simulink model "s4"  (Simulink 2.00)
settings: Solver=ode15s  StartTime=0.0  StopTime=tstop  MaxStep=0.1  RelTol=1e-6  AbsTol=1e-6
values from neighbouring files (symbols this model uses):
  AEx = 0.0012    [I3ESSR.M]    (also in SET1.M)
  BEx = 1.264    [I3ESSR.M]    (also in SET1.M)
  delio = x(3)    [M1.M]    (also in M3.M = delta4; M3G.M = delta4; M4.M = delta)
  Domega = 0    [I3ESSR.M]    (also in M3.M; M3G.M; M5.M = 1; SET1.M = 2)
  Dz = (rs+re)*(rs+re) + (xq+xe)*(xpd+xe)    [M1.M]    (also in M4.M = (re+rs)*(re+rs) + (xe + xq)*(xe + xpd))
  Edpo = x(2)    [M1.M]    (also in M4.M = Vdo - xpq*Iqo + rs*Ido)
  Efo = u(1)    [M1.M]    (also in M3.M = Eqo + (xd-xq)*Ido; M3G.M = Eqo + (xd-xq)*Ido; M4.M = Eqo + (xd-xq)*Ido)
  Eqpo = x(1)    [M1.M]    (also in M4.M = Vqo + xpd*Ido + rs*Iqo)
  H = 2.89    [I3ESSR.M]    (also in M1.M = 0.5*J_rotor*wbasem*wbasem/Sbase; M3.M = diag(h); M3G.M = diag(h); M5.M = 0.352825293175)
  KA = 50    [I3ESSR.M]    (also in SET1.M)
  KE = -0.0465    [I3ESSR.M]    (also in SET1.M)
  KF = 0.0832    [I3ESSR.M]    (also in SET1.M)
  Ks = 120    [M4.M]    (also in M4COMP.M)
  Pmecho = real(Sto)    [M4.M]
  pss_limit = 0.1    [M4.M]
  pss_sw = 5    [M4.M]
  re = 0.0    (= 0)    [M1.M]
  rs = 0.00    (= 0)    [I3ESSR.M]    (also in M1.M = rs/Zbase; M3.M; M3G.M = 0.001; M5.M = rs/Zb)
  T1 = 0.024    [M4.M]    (also in M4COMP.M)
  T2 = 0.002    [M4.M]    (also in M4COMP.M)
  T3 = 0.024    [M4.M]    (also in M4COMP.M)
  T4 = 0.24    [M4.M]    (also in M4COMP.M)
  TA = .06    (= 0.06)    [I3ESSR.M]    (also in SET1.M)
  TE = 0.052    [I3ESSR.M]    (also in SET1.M)
  TF = 1.0    (= 1)    [I3ESSR.M]    (also in SET1.M)
  Tpdo = 4.3    [I3ESSR.M]    (also in SET1.M = 7.9)
  Tpqo = 0.85    [I3ESSR.M]    (also in SET1.M = 0.41)
  Tw = 1.    (= 1)    [M4.M]    (also in M4COMP.M)
  Vio = abs(Vi)    [M4.M]
  VR = KE*Efo    [M4.M]
  Vref = abs(Vto)    [M4.M]
  VRmax = 1    [I3ESSR.M]    (also in SET1.M)
  VRmin = -1    [I3ESSR.M]    (also in SET1.M)
  Vs = Efo*KF/TF    [M4.M]
  wb = wbase    [M1.M]    (also in M2.M = 376.991118431; M3.M = 376.991118431; M3G.M = 376.991118431; M4.M = we)
  we = 2*pi*Frated    [M1.M]    (also in M4.M; M5.M = 710.48)
  xe = 0.0    (= 0)    [M1.M]    (also in M4.M = 0.1)
  xpd = 0.169    [I3ESSR.M]    (also in M1.M = xpd/Zbase; SET1.M = 0.355)
  xq = 1.71    [I3ESSR.M]    (also in M1.M = xq/Zbase; M3.M; M3G.M; M5.M = xq/Zb)
settings Model: SaveTime=off  SaveOutput=off  ConsistencyChecking=off

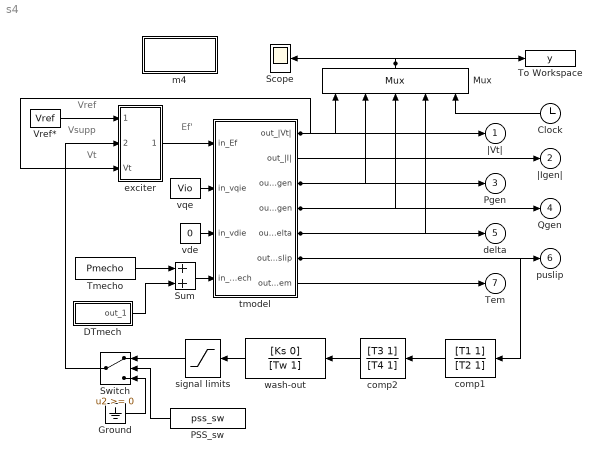
== system s4 ==
  note: Ef'
  note: Vsupp
  note: Vt
  note: Vref
  Clock : Clock
      settings: DeleteFcn=simclock BlockIsBeingDestroyed  PostSaveFcn=simclock Save
  DTmech : Subsystem  mask(Repeating table){@1=time_Dtmech, @2=tmech_Dtmech}
      mask prompts: @1 "Time values:"; @2 "Output values:"
      mask help:
      | Repeating table.
      | Enter values of time and output for first cycle.
      mask init:
      | period = max(@1); t = @1; y = @2;
      mask Help: Repeats cycle given in table. Time values should be monotonically increasing.
      mask Display: plot([t,t+period,t+2*period],[y,y,y])
  Ground : Ground
  m4 : Subsystem
      settings: OpenFcn=m4
      mask Type: Masked block of m4.m
      mask Help: Uses m4.m to initialize and plot
      mask Display: disp('Initialize\nand plot')
  Mux : Mux  Orientation=up  Inputs=5
  PSS_sw : Constant  Orientation=left  Value=pss_sw
  Scope : Scope
      settings: TickLabels=on  TimeRange=30  YMin=-2  YMax=2  SaveToWorkspace=off  SaveName=ScopeData  LimitMaxRows=off
  Sum : Sum  Inputs=++
  Switch : Switch  Orientation=left  Threshold=0
  Tmecho : Constant  Value=Pmecho
  To Workspace : ToWorkspace  VariableName=y  SampleTime=0
      settings: Buffer=10000
  Vref* : Constant  Value=Vref
  comp1 : TransferFcn  Orientation=left  Numerator=[T1 1]  Denominator=[T2 1]
  comp2 : TransferFcn  Orientation=left  Numerator=[T3 1]  Denominator=[T4 1]
  exciter : Subsystem
  signal limits : Saturate  Orientation=left  UpperLimit=pss_limit  LowerLimit=-pss_limit
  tmodel : Subsystem
  vde : Constant  Value=0
  vqe : Constant  Value=Vio
  wash-out : TransferFcn  Orientation=left  Numerator=[Ks 0]  Denominator=[Tw 1]
  |Vt| : Outport  Port=1  InitialOutput=0
  |Igen| : Outport  Port=2  InitialOutput=0
  Pgen : Outport  Port=3  InitialOutput=0
  Qgen : Outport  Port=4  InitialOutput=0
  delta : Outport  Port=5  InitialOutput=0
  puslip : Outport  Port=6  InitialOutput=0
  Tem : Outport  Port=7  InitialOutput=0
  wires:
  vqe/1 -> tmodel/2(in_vqie)
  vde/1 -> tmodel/3(in_vdie)
  tmodel/7(out_Tem) -> Tem/1
  tmodel/2(out_|I|) -> |Igen|/1
  Mux/1 -> Scope/1, To Workspace/1
  tmodel/1(out_|Vt|) -> |Vt|/1, Mux/1, exciter/3(Vt)
  exciter/1(out_Ef) -> tmodel/1(in_Ef)
  comp2/1 -> wash-out/1
  comp1/1 -> comp2/1
  tmodel/6(out_puslip) -> puslip/1, comp1/1
  wash-out/1 -> signal limits/1
  signal limits/1 -> Switch/1
  Switch/1 -> exciter/2(Vsupp)
  PSS_sw/1 -> Switch/2
  Vref*/1 -> exciter/1(Vref)
  Tmecho/1 -> Sum/1
  Sum/1 -> tmodel/4(in_Tmech)
  tmodel/3(out_Pgen) -> Pgen/1, Mux/2
  tmodel/4(out_Qgen) -> Qgen/1, Mux/3
  tmodel/5(out_delta) -> delta/1, Mux/4
  Clock/1 -> Mux/5
  DTmech/1(out_1) -> Sum/2
  Ground/1 -> Switch/3

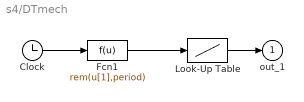
== system s4/DTmech ==
  Clock : Clock
      settings: DeleteFcn=simclock BlockIsBeingDestroyed  PostSaveFcn=simclock Save
  Fcn1 : Fcn  Expr=rem(u[1],period)
  Look-Up Table : Lookup  InputValues=t  OutputValues=y
  out_1 : Outport  Port=1  InitialOutput=0
  wires:
  Look-Up Table/1 -> out_1/1
  Clock/1 -> Fcn1/1
  Fcn1/1 -> Look-Up Table/1

== system s4/m4 ==
  note: Masked block of m4.m to initialize
      | s4.m in chapter 10 and to plot results

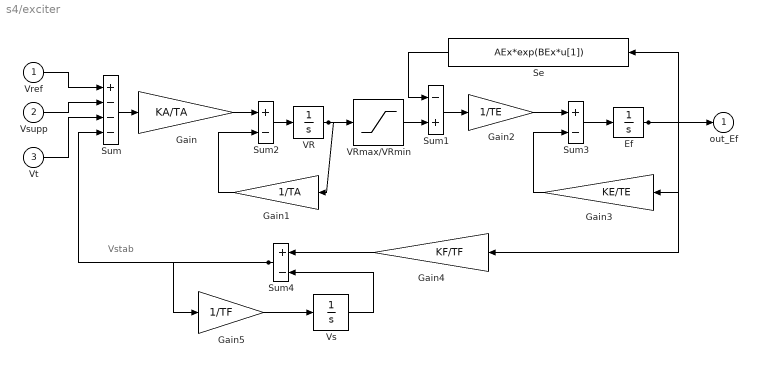
== system s4/exciter ==
  note: Vstab
  Vref : Inport  Port=1  PortWidth=-1  SampleTime=-1
  Vsupp : Inport  Port=2  PortWidth=-1  SampleTime=-1
  Vt : Inport  Port=3  PortWidth=-1  SampleTime=-1
  Ef : Integrator  ExternalReset=none  InitialConditionSource=internal  InitialCondition=Efo  LimitOutput=off  UpperSaturationLimit=inf  LowerSaturationLimit=-inf  ShowSaturationPort=off  ShowStatePort=off  AbsoluteTolerance=auto
  Gain : Gain  Gain=KA/TA
  Gain1 : Gain  Orientation=left  Gain=1/TA
  Gain2 : Gain  Gain=1/TE
  Gain3 : Gain  Orientation=left  Gain=KE/TE
  Gain4 : Gain  Orientation=left  Gain=KF/TF
  Gain5 : Gain  Gain=1/TF
  Se : Fcn  Orientation=left  Expr=AEx*exp(BEx*u[1])
  Sum : Sum  Inputs=+---
  Sum1 : Sum  Inputs=-+
  Sum2 : Sum  Inputs=+-
  Sum3 : Sum  Inputs=+-
  Sum4 : Sum  Orientation=left  Inputs=+-
  VR : Integrator  ExternalReset=none  InitialConditionSource=internal  InitialCondition=VR  LimitOutput=off  UpperSaturationLimit=inf  LowerSaturationLimit=-inf  ShowSaturationPort=off  ShowStatePort=off  AbsoluteTolerance=auto
  VRmax/VRmin : Saturate  UpperLimit=VRmax  LowerLimit=VRmin
  Vs : Integrator  ExternalReset=none  InitialConditionSource=internal  InitialCondition=Vs  LimitOutput=off  UpperSaturationLimit=inf  LowerSaturationLimit=-inf  ShowSaturationPort=off  ShowStatePort=off  AbsoluteTolerance=auto
  out_Ef : Outport  Port=1  InitialOutput=0
  wires:
  VRmax/VRmin/1 -> Sum1/2
  Vref/1 -> Sum/1
  Se/1 -> Sum1/1
  Sum2/1 -> VR/1
  Sum/1 -> Gain/1
  VR/1 -> VRmax/VRmin/1, Gain1/1
  Sum3/1 -> Ef/1
  Sum1/1 -> Gain2/1
  Gain2/1 -> Sum3/1
  Gain3/1 -> Sum3/2
  Ef/1 -> Gain3/1, Se/1, out_Ef/1, Gain4/1
  Gain/1 -> Sum2/1
  Gain1/1 -> Sum2/2
  Gain4/1 -> Sum4/1
  Gain5/1 -> Vs/1
  Vs/1 -> Sum4/2
  Sum4/1 -> Gain5/1, Sum/4
  Vt/1 -> Sum/3
  Vsupp/1 -> Sum/2

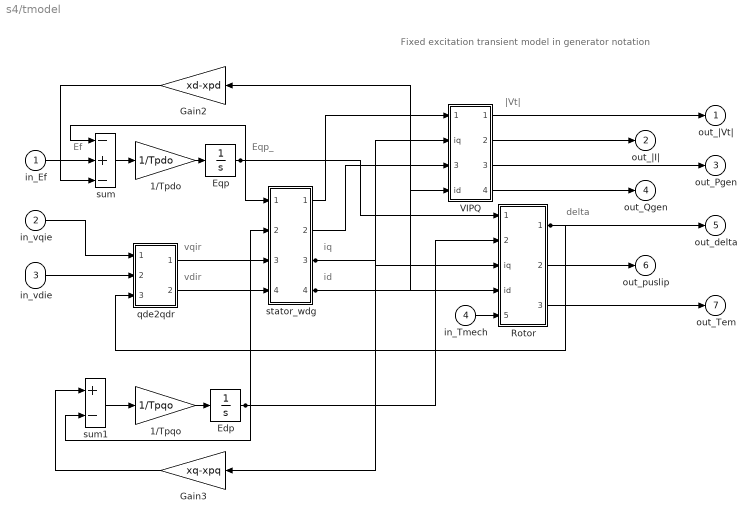
== system s4/tmodel ==
  note: Fixed excitation transient model in generator notation
  note: |Vt|
  note: id
  note: iq
  note: delta
  note: Ef
  note: vdir
  note: vqir
  note: Eqp_
  in_Ef : Inport  Port=1  PortWidth=-1  SampleTime=-1
  in_vqie : Inport  Port=2  PortWidth=-1  SampleTime=-1
  in_vdie : Inport  Port=3  PortWidth=-1  SampleTime=-1
  in_Tmech : Inport  Port=4  PortWidth=-1  SampleTime=-1
  1/Tpdo : Gain  Gain=1/Tpdo
  1/Tpqo : Gain  Gain=1/Tpqo
  Edp : Integrator  ExternalReset=none  InitialConditionSource=internal  InitialCondition=Edpo  LimitOutput=off  UpperSaturationLimit=inf  LowerSaturationLimit=-inf  ShowSaturationPort=off  ShowStatePort=off  AbsoluteTolerance=auto
  Eqp : Integrator  ExternalReset=none  InitialConditionSource=internal  InitialCondition=Eqpo  LimitOutput=off  UpperSaturationLimit=inf  LowerSaturationLimit=-inf  ShowSaturationPort=off  ShowStatePort=off  AbsoluteTolerance=auto
  Gain2 : Gain  Orientation=left  Gain=xd-xpd
  Gain3 : Gain  Orientation=left  Gain=xq-xpq
  Rotor : Subsystem
  VIPQ : Subsystem
  qde2qdr : Subsystem
  stator_wdg : Subsystem
  sum : Sum  Inputs=-+-
  sum1 : Sum  Inputs=+-
  out_|Vt| : Outport  Port=1  InitialOutput=0
  out_|I| : Outport  Port=2  InitialOutput=0
  out_Pgen : Outport  Port=3  InitialOutput=0
  out_Qgen : Outport  Port=4  InitialOutput=0
  out_delta : Outport  Port=5  InitialOutput=0
  out_puslip : Outport  Port=6  InitialOutput=0
  out_Tem : Outport  Port=7  InitialOutput=0
  wires:
  Eqp/1 -> stator_wdg/1(Eqp), Rotor/1(Eqp), sum/1
  1/Tpdo/1 -> Eqp/1
  sum/1 -> 1/Tpdo/1
  Gain2/1 -> sum/3
  VIPQ/2(out_|I|) -> out_|I|/1
  VIPQ/3(out_P) -> out_Pgen/1
  VIPQ/4(out_Q) -> out_Qgen/1
  Rotor/1(out_delta) -> qde2qdr/3("delta "), out_delta/1
  Rotor/2(out_puslip) -> out_puslip/1
  in_vqie/1 -> qde2qdr/1(vqe)
  in_vdie/1 -> qde2qdr/2(vde)
  stator_wdg/1(out_vqt) -> VIPQ/1(vqt)
  stator_wdg/2(out_vdt) -> VIPQ/3(vdt)
  stator_wdg/4(out_id) -> VIPQ/4(id), Gain2/1, Rotor/4(id)
  in_Ef/1 -> sum/2
  Rotor/3(Tem) -> out_Tem/1
  1/Tpqo/1 -> Edp/1
  sum1/1 -> 1/Tpqo/1
  stator_wdg/3(out_iq) -> VIPQ/2(iq), Gain3/1, Rotor/3(iq)
  Gain3/1 -> sum1/1
  Edp/1 -> sum1/2, stator_wdg/2(Edp), Rotor/2(Edp)
  qde2qdr/1(vqr) -> stator_wdg/3(vqir)
  qde2qdr/2(vdr) -> stator_wdg/4(vdir)
  in_Tmech/1 -> Rotor/5(T_mech)
  VIPQ/1(out_|Vt|) -> out_|Vt|/1

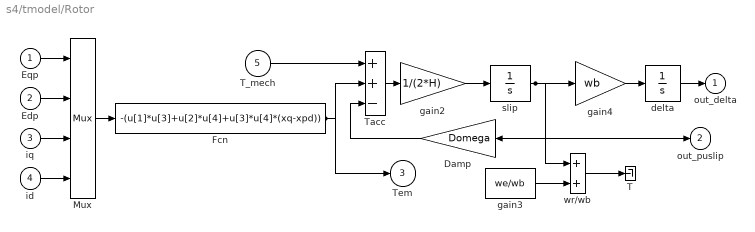
== system s4/tmodel/Rotor ==
  Eqp : Inport  Port=1  PortWidth=-1  SampleTime=-1
  Edp : Inport  Port=2  PortWidth=-1  SampleTime=-1
  iq : Inport  Port=3  PortWidth=-1  SampleTime=-1
  id : Inport  Port=4  PortWidth=-1  SampleTime=-1
  T_mech : Inport  Port=5  PortWidth=-1  SampleTime=-1
  Damp : Gain  Orientation=left  Gain=Domega
  Fcn : Fcn  Expr=-(u[1]*u[3]+u[2]*u[4]+u[3]*u[4]*(xq-xpd))
  Mux : Mux  Inputs=4
  T : Terminator
  Tacc : Sum  Inputs=++-
  delta : Integrator  ExternalReset=none  InitialConditionSource=internal  InitialCondition=delio  LimitOutput=off  UpperSaturationLimit=inf  LowerSaturationLimit=-inf  ShowSaturationPort=off  ShowStatePort=off  AbsoluteTolerance=auto
  gain2 : Gain  Gain=1/(2*H)
  gain3 : Constant  Value=we/wb
  gain4 : Gain  Gain=wb
  slip : Integrator  ExternalReset=none  InitialConditionSource=internal  InitialCondition=0  LimitOutput=off  UpperSaturationLimit=inf  LowerSaturationLimit=-inf  ShowSaturationPort=off  ShowStatePort=off  AbsoluteTolerance=auto
  wr/wb : Sum  Inputs=++
  out_delta : Outport  Port=1  InitialOutput=0
  out_puslip : Outport  Port=2  InitialOutput=0
  Tem : Outport  Port=3  InitialOutput=0
  wires:
  Damp/1 -> Tacc/3
  T_mech/1 -> Tacc/1
  delta/1 -> out_delta/1
  Tacc/1 -> gain2/1
  gain3/1 -> wr/wb/2
  gain2/1 -> slip/1
  gain4/1 -> delta/1
  slip/1 -> wr/wb/1, gain4/1, Damp/1, out_puslip/1
  Fcn/1 -> Tacc/2, Tem/1
  Mux/1 -> Fcn/1
  Eqp/1 -> Mux/1
  iq/1 -> Mux/3
  id/1 -> Mux/4
  Edp/1 -> Mux/2
  wr/wb/1 -> T/1

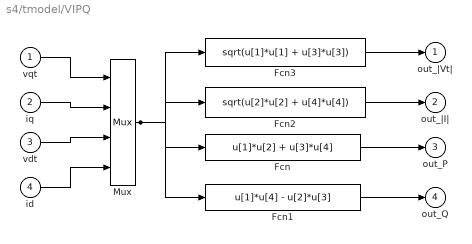
== system s4/tmodel/VIPQ ==
  vqt : Inport  Port=1  PortWidth=-1  SampleTime=-1
  iq : Inport  Port=2  PortWidth=-1  SampleTime=-1
  vdt : Inport  Port=3  PortWidth=-1  SampleTime=-1
  id : Inport  Port=4  PortWidth=-1  SampleTime=-1
  Fcn : Fcn  Expr=u[1]*u[2] + u[3]*u[4]
  Fcn1 : Fcn  Expr=u[1]*u[4] - u[2]*u[3]
  Fcn2 : Fcn  Expr=sqrt(u[2]*u[2] + u[4]*u[4])
  Fcn3 : Fcn  Expr=sqrt(u[1]*u[1] + u[3]*u[3])
  Mux : Mux  Inputs=4
  out_|Vt| : Outport  Port=1  InitialOutput=0
  out_|I| : Outport  Port=2  InitialOutput=0
  out_P : Outport  Port=3  InitialOutput=0
  out_Q : Outport  Port=4  InitialOutput=0
  wires:
  vqt/1 -> Mux/1
  iq/1 -> Mux/2
  vdt/1 -> Mux/3
  id/1 -> Mux/4
  Fcn/1 -> out_P/1
  Fcn1/1 -> out_Q/1
  Mux/1 -> Fcn/1, Fcn1/1, Fcn3/1, Fcn2/1
  Fcn3/1 -> out_|Vt|/1
  Fcn2/1 -> out_|I|/1

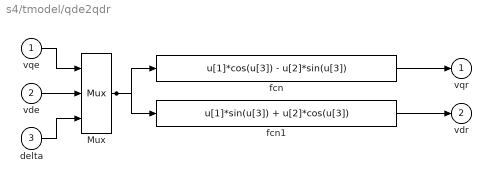
== system s4/tmodel/qde2qdr ==
  vqe : Inport  Port=1  PortWidth=-1  SampleTime=-1
  vde : Inport  Port=2  PortWidth=-1  SampleTime=-1
  "delta " : Inport  Port=3  PortWidth=-1  SampleTime=-1
  Mux : Mux  Inputs=3
  fcn : Fcn  Expr=u[1]*cos(u[3]) - u[2]*sin(u[3])
  fcn1 : Fcn  Expr=u[1]*sin(u[3]) + u[2]*cos(u[3])
  vqr : Outport  Port=1  InitialOutput=0
  vdr : Outport  Port=2  InitialOutput=0
  wires:
  fcn1/1 -> vdr/1
  vqe/1 -> Mux/1
  fcn/1 -> vqr/1
  Mux/1 -> fcn/1, fcn1/1
  "delta "/1 -> Mux/3
  vde/1 -> Mux/2

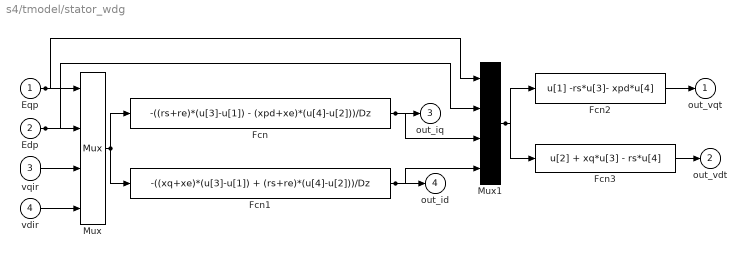
== system s4/tmodel/stator_wdg ==
  Eqp : Inport  Port=1  PortWidth=-1  SampleTime=-1
  Edp : Inport  Port=2  PortWidth=-1  SampleTime=-1
  vqir : Inport  Port=3  PortWidth=-1  SampleTime=-1
  vdir : Inport  Port=4  PortWidth=-1  SampleTime=-1
  Fcn : Fcn  Expr=-((rs+re)*(u[3]-u[1]) - (xpd+xe)*(u[4]-u[2]))/Dz
  Fcn1 : Fcn  Expr=-((xq+xe)*(u[3]-u[1]) + (rs+re)*(u[4]-u[2]))/Dz
  Fcn2 : Fcn  Expr=u[1] -rs*u[3]- xpd*u[4]
  Fcn3 : Fcn  Expr=u[2] + xq*u[3] - rs*u[4]
  Mux : Mux  Inputs=4
  Mux1 : Mux  Inputs=4
  out_vqt : Outport  Port=1  InitialOutput=0
  out_vdt : Outport  Port=2  InitialOutput=0
  out_iq : Outport  Port=3  InitialOutput=0
  out_id : Outport  Port=4  InitialOutput=0
  wires:
  Mux/1 -> Fcn/1, Fcn1/1
  Mux1/1 -> Fcn2/1, Fcn3/1
  Fcn2/1 -> out_vqt/1
  Fcn3/1 -> out_vdt/1
  vqir/1 -> Mux/3
  vdir/1 -> Mux/4
  Fcn1/1 -> out_id/1, Mux1/4
  Fcn/1 -> out_iq/1, Mux1/3
  Eqp/1 -> Mux/1, Mux1/1
  Edp/1 -> Mux/2, Mux1/2
